simulink subsystem "Final_Project_PreBusUnpack_20260601_105527"  (R2024a)
settings: Solver=VariableStepAuto  StartTime=0.0  StopTime=10.0  RelTol=1e-3
values from neighbouring files (symbols this model uses):
  D = hypot(Ep(:,1)-Tp(:,1)',Ep(:,2)-Tp(:,2)')    [pp_compare_stage.m]    (also in pp_diag_path.m; pp_t09_clear.m = hypot(Ep(:,1)-Tperim(:,1)', Ep(:,2)-Tperim(:,2)'); pp_tune2.m)
undefined symbols (not defined in the file or in its folder): waypoints
libraries: CarMaker4SL x116, simulink x1
(part 5 of 7)

== matlab function Final_Project_PreBusUnpack_20260601_105527/Driving_Module_Ver.3_PSH/Subsystem/Controller ==
  data: ego_cross_track_err input; steer output; ego_head_err input; ego_max_curvature input; target_speed input; lead_dist input; lead_speed input; drive_state input; lane_settled input; submission_state input; ego_state input; accel output; front_dist_lock output; gear_pos output
function [steer, accel, front_dist_lock, gear_pos] = controller(...
    ego_cross_track_err, ego_head_err, ego_max_curvature, target_speed, ...
    lead_dist, lead_speed, drive_state, lane_settled, submission_state, ego_state)
%#codegen

    % ============================================================
    % 기본 상수
    % ============================================================
    TS           = 0.01;
    STEER_LIM    = 0.58;
    MAX_SPEED    = 50.0;
    MODE_LCHG    = int32(1);
    MODE_PARK    = int32(2);
    KAPPA_EPS    = 1e-4;
    SPD_DEADBAND = 0.3;

    % ============================================================
    % Ego unpack
    % ============================================================
    ego_x = ego_state.Car_Fr1_tx;
    ego_y = ego_state.Car_Fr1_ty;
    ego_v = ego_state.Ego_V;

    % ============================================================
    % Parking waypoints
    % ============================================================
    L4_X     = -46.856;  L4_Y     = 15.842;
    L5_END_X =  2.617;   L5_END_Y = -35.0;

    dist_l4     = sqrt((ego_x - L4_X)^2     + (ego_y - L4_Y)^2);
    dist_to_end = sqrt((ego_x - L5_END_X)^2 + (ego_y - L5_END_Y)^2);

    % ============================================================
    % 파라미터 정의: 일반 주행 / 주차 진입
    % ============================================================
    K_STANLEY_NRM  = 0.88;   K_STANLEY_PRK  = 0.20;
    KP_HEAD_NRM    = 0.90;   KP_HEAD_PRK    = 0.50;
    LOOK_FRONT_NRM = calcLookFront(ego_v);  LOOK_FRONT_PRK = 10.0;
    ALAT_NRM       = 3.50;   ALAT_PRK       = 1.50;
    ATOT_NRM       = 4.00;   ATOT_PRK       = 2.00;
    MCSPD_NRM      = 7.00;   MCSPD_PRK      = 1.00;
    VREF_A_NRM     = 50.0;   VREF_A_PRK     = 2.00;
    VREF_D_NRM     = 100.0;  VREF_D_PRK     = 5.00;
    JERK_U_NRM     = 50.0;   JERK_U_PRK     = 3.00;
    JERK_D_NRM     = 60.0;   JERK_D_PRK     = 5.00;
    AMAX_NRM       = 10.0;   AMAX_PRK       = 3.00;
    DMAX_NRM       = 10.0;   DMAX_PRK       = 5.00;

    % ============================================================
    % park_cmd에 따른 파라미터 보간
    % L4에 가까워질수록 일반 주행 -> 주차 진입 파라미터로 전환
    % ============================================================
    FADE_FAR  = 50.0;
    FADE_NEAR = 20.0;

    if submission_state == int32(1)
        if dist_l4 >= FADE_FAR
            r = 0.0;
        elseif dist_l4 <= FADE_NEAR
            r = 1.0;
        else
            r = (FADE_FAR - dist_l4) / (FADE_FAR - FADE_NEAR);
        end
    else
        r = 0.0;
    end

    K_STANLEY       = K_STANLEY_NRM  + r * (K_STANLEY_PRK  - K_STANLEY_NRM);
    KP_HEAD         = KP_HEAD_NRM    + r * (KP_HEAD_PRK    - KP_HEAD_NRM);
    LOOK_FRONT      = LOOK_FRONT_NRM + r * (LOOK_FRONT_PRK - LOOK_FRONT_NRM);
    A_LAT_LIMIT     = ALAT_NRM       + r * (ALAT_PRK       - ALAT_NRM);
    A_TOTAL_LIMIT   = ATOT_NRM       + r * (ATOT_PRK       - ATOT_NRM);
    MIN_CURVE_SPEED = MCSPD_NRM      + r * (MCSPD_PRK      - MCSPD_NRM);
    V_REF_ACCEL     = VREF_A_NRM     + r * (VREF_A_PRK     - VREF_A_NRM);
    V_REF_DECEL     = VREF_D_NRM     + r * (VREF_D_PRK     - VREF_D_NRM);
    JERK_UP         = JERK_U_NRM     + r * (JERK_U_PRK     - JERK_U_NRM);
    JERK_DOWN       = JERK_D_NRM     + r * (JERK_D_PRK     - JERK_D_NRM);
    ACCEL_MAX_BASE  = AMAX_NRM       + r * (AMAX_PRK       - AMAX_NRM);
    DECEL_MAX_BASE  = DMAX_NRM       + r * (DMAX_PRK       - DMAX_NRM);

    % ============================================================
    % L4 통과 latch
    % ============================================================
    persistent l4_passed_p l4_pass_init_p

    if isempty(l4_pass_init_p)
        l4_passed_p    = false;
        l4_pass_init_p = true;
    end

    if submission_state ~= int32(1)
        l4_passed_p = false;
    end

    L4_PASS_DIST = 3.0;

    if submission_state == int32(1) && dist_l4 < L4_PASS_DIST
        l4_passed_p = true;
    end

    % ============================================================
    % 목표속도 결정
    % ============================================================
    if submission_state == int32(1)

        DECEL_DIST = 25.0;
        STOP_DIST  =  2.0;

        SPD_BEFORE_L4_FAR  = 12.3;
        SPD_BEFORE_L4_NEAR = 4.8;
        SPD_AFTER_L4       = 5.8;
        SPD_PARK_INSIDE    = 4.2;

        if drive_state == MODE_PARK

            if dist_to_end < STOP_DIST
                ts = 0.0;
            elseif dist_to_end < DECEL_DIST
                ts = SPD_PARK_INSIDE * (dist_to_end / DECEL_DIST);
            else
                ts = SPD_PARK_INSIDE;
            end

        elseif l4_passed_p

            ts = SPD_AFTER_L4;

        elseif dist_l4 > FADE_NEAR

            if dist_l4 >= FADE_FAR
                ts = SPD_BEFORE_L4_FAR;
            else
                ts = SPD_BEFORE_L4_FAR + ...
                     (SPD_BEFORE_L4_NEAR - SPD_BEFORE_L4_FAR) * r;
            end

        else

            ts = SPD_AFTER_L4;

        end

    else

        ts = target_speed;

        if ts > 20.0
            ts = ts / 3.6;
        end

    end

    if ts > MAX_SPEED
        ts = MAX_SPEED;
    end

    if ts < 0.0
        ts = 0.0;
    end

    % ============================================================
    % persistent
    % ============================================================
    persistent desired_v_p accel_p did_init

    if isempty(did_init)
        desired_v_p = ego_v;
        accel_p     = 0.0;
        did_init    = true;
    end

    % ============================================================
    % 1. Stanley 조향
    % ============================================================
    v_safe = ego_v;

    if v_safe < 1.0
        v_safe = 1.0;
    end

    steer = KP_HEAD * ego_head_err - atan2(K_STANLEY * ego_cross_track_err, v_safe);

    if steer > STEER_LIM
        steer = STEER_LIM;
    elseif steer < -STEER_LIM
        steer = -STEER_LIM;
    end

    % ============================================================
    % 1-1. 끝점 추가 좌회전 블렌드
    % submission_state=1, MODE_PARK, 끝점 5m 이내에서만 적용
    % ============================================================
    EXTRA_DIST = 5.0;
    EXTRA_RAD  = pi / 3.0;

    if submission_state == int32(1) && drive_state == MODE_PARK
        if dist_to_end < EXTRA_DIST && dist_to_end > 0.0
            blend = 1.0 - (dist_to_end / EXTRA_DIST);
            steer = steer + blend * EXTRA_RAD;

            if steer > EXTRA_RAD
                steer = EXTRA_RAD;
            elseif steer < -EXTRA_RAD
                steer = -EXTRA_RAD;
            end
        end
    end

    % ============================================================
    % 2. 곡률 기반 목표속도 제한
    % ============================================================
    desired_v_raw = ts;

    if ego_max_curvature > KAPPA_EPS

        v_curve = sqrt(A_LAT_LIMIT / ego_max_curvature);

        if v_curve < MIN_CURVE_SPEED
            v_curve = MIN_CURVE_SPEED;
        end

        if v_curve < desired_v_raw
            desired_v_raw = v_curve;
        end
    end

    % ============================================================
    % 3. ACC 앞차 감속
    % MODE_PARK 전까지는 앞차 감속 적용
    % ============================================================
    if drive_state ~= MODE_PARK

        if lead_dist < LOOK_FRONT

            time_gap = 2.0;
            ACC_GAIN = 0.5;

            safe_v = lead_speed + (lead_dist - time_gap * ego_v) * ACC_GAIN;

            if safe_v < desired_v_raw
                desired_v_raw = safe_v;
            end
        end
    end

    if desired_v_raw < 0.0
        desired_v_raw = 0.0;
    end

    % ============================================================
    % 4. 목표속도 변화율 제한
    % ============================================================
    dv = desired_v_raw - desired_v_p;

    max_dv_up = V_REF_ACCEL * TS;
    max_dv_dn = V_REF_DECEL * TS;

    if dv > max_dv_up
        desired_v_p = desired_v_p + max_dv_up;
    elseif dv < -max_dv_dn
        desired_v_p = desired_v_p - max_dv_dn;
    else
        desired_v_p = desired_v_raw;
    end

    desired_v = desired_v_p;

    % ============================================================
    % 5. 가감속
    % 주차 구간: 비례제어
    % 일반 구간: 기록 단축용 Bang-Bang
    % ============================================================
    spd_err = desired_v - ego_v;

    if submission_state == int32(1)

        KP_SPD = 2.0;
        accel_cmd = KP_SPD * spd_err;

        if accel_cmd > ACCEL_MAX_BASE
            accel_cmd = ACCEL_MAX_BASE;
        elseif accel_cmd < -DECEL_MAX_BASE
            accel_cmd = -DECEL_MAX_BASE;
        end

    else

        if spd_err > SPD_DEADBAND
            accel_cmd = ACCEL_MAX_BASE;
        elseif spd_err < -SPD_DEADBAND
            accel_cmd = -DECEL_MAX_BASE;
        else
            accel_cmd = 0.5 * spd_err;
        end

    end

    % ============================================================
    % 6. Friction circle 기반 가속 한계
    % ============================================================
    a_lat_now = ego_v * ego_v * ego_max_curvature;

    if a_lat_now >= A_TOTAL_LIMIT
        a_lon_avail = 0.5;
    else
        a_lon_avail = sqrt(A_TOTAL_LIMIT * A_TOTAL_LIMIT - a_lat_now * a_lat_now);

        if a_lon_avail < 0.5
            a_lon_avail = 0.5;
        end
    end

    accel_max = ACCEL_MAX_BASE;

    if a_lon_avail < accel_max
        accel_max = a_lon_avail;
    end

    if accel_cmd > accel_max
        accel_cmd = accel_max;
    end

    if accel_cmd < -DECEL_MAX_BASE
        accel_cmd = -DECEL_MAX_BASE;
    end

    % ============================================================
    % 7. Jerk 제한
    % ============================================================
    da = accel_cmd - accel_p;

    max_da_up = JERK_UP   * TS;
    max_da_dn = JERK_DOWN * TS;

    if da > max_da_up
        accel_p = accel_p + max_da_up;
    elseif da < -max_da_dn
        accel_p = accel_p - max_da_dn;
    else
        accel_p = accel_cmd;
    end

    accel = accel_p;

    % ============================================================
    % 8. front_dist_lock
    % ============================================================
    if drive_state == MODE_LCHG || lane_settled
        front_dist_lock = 0;
    else
        front_dist_lock = lead_dist;
    end

    % ============================================================
    % 9. Gear Position
    % 1 : Drive
    % ============================================================
    gear_pos = int32(1);

end


function LOOK_FRONT = calcLookFront(v)
%#codegen

    v = abs(v);

    if v > 60.0
        v = v / 3.6;
    end

    V_HIGH = 80.0 / 3.6;

    if v < V_HIGH
        LOOK_FRONT = 25.0 + 1.0 * v;
    else
        LOOK_FRONT = 50.0 + 1.0 * V_HIGH + 30.0 * (v - V_HIGH);
    end

    if LOOK_FRONT > 120.0
        LOOK_FRONT = 120.0;
    end

end

== matlab function Final_Project_PreBusUnpack_20260601_105527/MATLAB Function3 ==
  settings: sampleTime=0.1
  data: map input size=[200 200]; y output size=[200 200]; traffic_info input; traffic_size input
function y = add_obstacle_(map, traffic_info, traffic_size)
%ADD_OBSTACLE_ Build a half-width-inflated binary occupancy map.
%
%   y = add_obstacle_(map, traffic_info, traffic_size)
%
%   traffic_info is CarMaker Traffic.StartPos [x;y;yaw] repeated for T00..T20.
%   traffic_size is [width; length].
%   The ego/path state is rear-bumper based, but CarMaker traffic StartPos is
%   the traffic-object reference point near the box center, not the rear bumper.
%
%#codegen

u = map(1, 1) * 0 + traffic_info(1) * 0 + traffic_size(1) * 0;

persistent cached_occ cached_init
if isempty(cached_init)
    cached_occ = double(add_obstacle_local(uint8(map), traffic_info, traffic_size));
    cached_init = true;
end

y = cached_occ + u;
end

function occ = add_obstacle_local(base_map, traffic_info, traffic_size)
%#codegen
c = map_const_local();
N = c.N;
res = c.RES;
x_min = c.X_MIN;
y_max = c.Y_MAX;

veh_w = traffic_size(1);
veh_l = traffic_size(2);

static_map = base_map;

num_traffic = int32(floor(double(numel(traffic_info)) / 3.0));
if num_traffic > int32(21)
    num_traffic = int32(21);
end

for i = 1:num_traffic
    idx = (i - 1) * 3;
    ref_x = traffic_info(idx + 1);
    ref_y = traffic_info(idx + 2);
    yaw    = traffic_info(idx + 3);

    if abs(ref_x) < 1.0e-6 && abs(ref_y) < 1.0e-6 && abs(yaw) < 1.0e-6
        continue;
    end

    c_yaw = cos(yaw);
    s_yaw = sin(yaw);

    half_w = veh_w * 0.5;
    pad = c.RES;
    x0 = 0.0;
    x1 = veh_l;
    xs = [x0, x0, x1, x1];
    ys = [-half_w, half_w, half_w, -half_w];
    wx_min =  1.0e18; wx_max = -1.0e18;
    wy_min =  1.0e18; wy_max = -1.0e18;
    for ci = 1:4
        wx_c = ref_x + xs(ci) * c_yaw - ys(ci) * s_yaw;
        wy_c = ref_y + xs(ci) * s_yaw + ys(ci) * c_yaw;
        if wx_c < wx_min; wx_min = wx_c; end
        if wx_c > wx_max; wx_max = wx_c; end
        if wy_c < wy_min; wy_min = wy_c; end
        if wy_c > wy_max; wy_max = wy_c; end
    end
    wx_min = wx_min - pad; wx_max = wx_max + pad;
    wy_min = wy_min - pad; wy_max = wy_max + pad;

    col_min = int32(floor((wx_min - x_min) / res)) + int32(1);
    col_max = int32(floor((wx_max - x_min) / res)) + int32(1);
    row_min = int32(floor((y_max - wy_max) / res)) + int32(1);
    row_max = int32(floor((y_max - wy_min) / res)) + int32(1);

    col_min = max(int32(1), col_min - int32(1));
    col_max = min(N,        col_max + int32(1));
    row_min = max(int32(1), row_min - int32(1));
    row_max = min(N,        row_max + int32(1));

    for row = row_min:row_max
        wy = y_max - (double(row) - 0.5) * res;
        for col = col_min:col_max
            wx = x_min + (double(col) - 0.5) * res;
            dx = wx - ref_x;
            dy = wy - ref_y;
            lx =  c_yaw * dx + s_yaw * dy;
            ly = -s_yaw * dx + c_yaw * dy;
            if lx >= x0 && lx <= x1 && abs(ly) <= half_w
                static_map(row, col) = uint8(1);
            end
        end
    end
end

% Adjacent parked cars often leave a mathematically free but physically unsafe
% slot gap. Treat those narrow side-by-side gaps as blocked so the planner does
% not try to squeeze an EV6 through spaces such as T00-T12 (~3.3 m clear).
static_map = close_side_by_side_gaps(static_map, traffic_info, traffic_size);

% Keep obstacle inflation modest; ego width is handled by the planner's
% swept-footprint collision checker.
inflate_r = c.CENTERLINE_SAFETY_BUFFER;
occ = inflate_binary_map(static_map, inflate_r);
end

function occ_map = close_side_by_side_gaps(occ_map, traffic_info, traffic_size)
%#codegen
c = map_const_local();
num_traffic = int32(floor(double(numel(traffic_info)) / 3.0));
if num_traffic > int32(21)
    num_traffic = int32(21);
end

for i = int32(1):num_traffic-int32(1)
    idx_i = (i - 1) * 3;
    xi = traffic_info(idx_i + 1);
    yi = traffic_info(idx_i + 2);
    yawi = traffic_info(idx_i + 3);
    if abs(xi) < 1.0e-6 && abs(yi) < 1.0e-6 && abs(yawi) < 1.0e-6
        continue;
    end
    [ix0, ix1, iy0, iy1] = vehicle_bbox(xi, yi, yawi, traffic_size);

    for j = i+int32(1):num_traffic
        idx_j = (j - 1) * 3;
        xj = traffic_info(idx_j + 1);
        yj = traffic_info(idx_j + 2);
        yawj = traffic_info(idx_j + 3);
        if abs(xj) < 1.0e-6 && abs(yj) < 1.0e-6 && abs(yawj) < 1.0e-6
            continue;
        end
        if abs(wrap_pi_local(yawi - yawj)) > 0.25
            continue;
        end

        [jx0, jx1, jy0, jy1] = vehicle_bbox(xj, yj, yawj, traffic_size);
        y_overlap = min(iy1, jy1) - max(iy0, jy0);
        if y_overlap < 2.5
            continue;
        end

        gap_x0 = 0.0;
        gap_x1 = 0.0;
        if ix1 < jx0
            gap_x0 = ix1;
            gap_x1 = jx0;
        elseif jx1 < ix0
            gap_x0 = jx1;
            gap_x1 = ix0;
        else
            continue;
        end

        gap_w = gap_x1 - gap_x0;
        if gap_w < 0.40 || gap_w > c.NARROW_GAP_BLOCK_MAX
            continue;
        end

        pad_x = c.NARROW_GAP_PAD_X;
        pad_y = c.NARROW_GAP_PAD_Y;
        x_min = gap_x0 - pad_x;
        x_max = gap_x1 + pad_x;
        y_min = max(iy0, jy0) - pad_y;
        y_max = min(iy1, jy1) + pad_y;
        occ_map = fill_world_rect(occ_map, x_min, x_max, y_min, y_max, c);
    end
end
end

function [wx_min, wx_max, wy_min, wy_max] = vehicle_bbox(ref_x, ref_y, yaw, traffic_size)
%#codegen
c = map_const_local();
veh_w = traffic_size(1);
veh_l = traffic_size(2);
c_yaw = cos(yaw);
s_yaw = sin(yaw);
half_w = veh_w * 0.5;
x0 = 0.0;
x1 = veh_l;
xs = [x0, x0, x1, x1];
ys = [-half_w, half_w, half_w, -half_w];
wx_min =  1.0e18; wx_max = -1.0e18;
wy_min =  1.0e18; wy_max = -1.0e18;
for k = 1:4
    wx = ref_x + xs(k) * c_yaw - ys(k) * s_yaw;
    wy = ref_y + xs(k) * s_yaw + ys(k) * c_yaw;
    if wx < wx_min; wx_min = wx; end
    if wx > wx_max; wx_max = wx; end
    if wy < wy_min; wy_min = wy; end
    if wy > wy_max; wy_max = wy; end
end
end

function occ_map = fill_world_rect(occ_map, x_min, x_max, y_min, y_max, c)
%#codegen
col_min = int32(floor((x_min - c.X_MIN) / c.RES)) + int32(1);
col_max = int32(floor((x_max - c.X_MIN) / c.RES)) + int32(1);
row_min = int32(floor((c.Y_MAX - y_max) / c.RES)) + int32(1);
row_max = int32(floor((c.Y_MAX - y_min) / c.RES)) + int32(1);
col_min = max(int32(1), col_min);
col_max = min(c.N, col_max);
row_min = max(int32(1), row_min);
row_max = min(c.N, row_max);
for row = row_min:row_max
    for col = col_min:col_max
        occ_map(row, col) = uint8(1);
    end
end
end

function a = wrap_pi_local(a)
%#codegen
while a > pi;  a = a - 2.0 * pi; end
while a < -pi; a = a + 2.0 * pi; end
end

function inflated = inflate_binary_map(occ_map, radius)
%#codegen
c = map_const_local();
inflated = uint8(occ_map);
rad_cells = int32(ceil(radius / c.RES));
r2 = radius * radius;

for row = int32(1):c.N
    for col = int32(1):c.N
        if occ_map(row, col) > 0
            r0 = max(int32(1), row - rad_cells);
            r1 = min(c.N, row + rad_cells);
            c0 = max(int32(1), col - rad_cells);
            c1 = min(c.N, col + rad_cells);
            for rr = r0:r1
                dy = double(rr - row) * c.RES;
                for cc = c0:c1
                    dx = double(cc - col) * c.RES;
                    if dx * dx + dy * dy <= r2
                        inflated(rr, cc) = uint8(1);
                    end
                end
            end
        end
    end
end
end

function c = map_const_local()
%#codegen
c.N        = int32(200);
c.RES      = 0.5;
c.X_MIN    = 0.0;
c.X_MAX    = 100.0;
c.Y_MIN    = -100.0;
c.Y_MAX    = 0.0;
c.TRUCK_W  = 2.48;
c.TRUCK_L  = 11.5;
c.EGO_W    = 1.9;
c.EGO_L    = 4.7;
c.WHEELBASE = 2.8;
c.TRAFFIC_BOX_X_OFFSET = 0.15;
c.SAFETY_MARGIN = 0.8;
c.CENTERLINE_SAFETY_BUFFER = 0.10;
c.NARROW_GAP_BLOCK_MAX = 4.20;
c.NARROW_GAP_PAD_X = 1.25;
c.NARROW_GAP_PAD_Y = 1.35;
c.CLEAR_MAX = 3.0;
c.W_CLEAR   = 1.2;
c.PARK_BOX_L = 6.0;
c.PARK_BOX_W = 3.0;
c.PARK_TOL   = 0.05;
end
